simulink model "passband_filter_2023b"  (R2023b)
settings: Solver=VariableStepAuto  StartTime=0.0  StopTime=10.768  RelTol=1e-3
values from neighbouring files (symbols this model uses):
  den = den{1}    [Km_con_filtri.m]    (also in fft_signal_analysis.m)
  den2 = den2{1}    [Km_con_filtri.m]    (also in fft_signal_analysis.m)
  num = num{1}    [Km_con_filtri.m]    (also in fft_signal_analysis.m)
  num2 = num2{1}    [Km_con_filtri.m]    (also in fft_signal_analysis.m)
settings Model: Creator=riccardoorlandi  LastModifiedBy=lollo
settings RTWCC: GPUComputeCapability=5.0

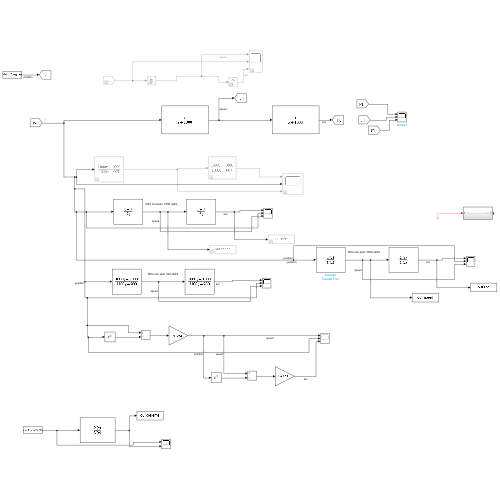
[thumbnail: Simulink's stored preview of the top-level diagram]
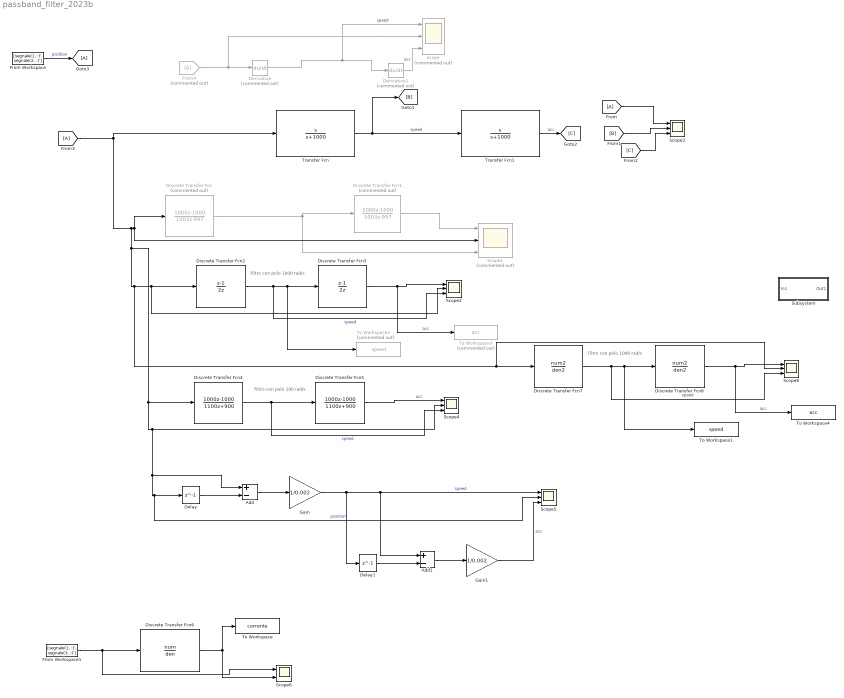
== system passband_filter_2023b ==
  note: filtro con polo 100 rad/s
  note: filtro con polo 1000 rad/s
  note: filtro con polo 1000 rad/s
  Add : Sum  Inputs=+-
  Add1 : Sum  Inputs=+-
  Delay : Delay  DelayLength=1
  Delay1 : Delay  DelayLength=1
  Derivative : Derivative  Commented=on
  Derivative1 : Derivative  Commented=on
  Discrete Transfer Fcn : DiscreteTransferFcn  Commented=on  Numerator=[1000 -1000]  Denominator=[1003 -997]
  Discrete Transfer Fcn1 : DiscreteTransferFcn  Commented=on  Numerator=[1000 -1000]  Denominator=[1003 -997]
  Discrete Transfer Fcn2 : DiscreteTransferFcn  Numerator=[1 -1]  Denominator=[2 0]
  Discrete Transfer Fcn3 : DiscreteTransferFcn  Numerator=[1 -1]  Denominator=[2 0]
  Discrete Transfer Fcn4 : DiscreteTransferFcn  Numerator=[1000 -1000]  Denominator=[1100 900]
  Discrete Transfer Fcn5 : DiscreteTransferFcn  Numerator=[1000 -1000]  Denominator=[1100 900]
  Discrete Transfer Fcn6 : DiscreteTransferFcn  Numerator=num  Denominator=den
  Discrete Transfer Fcn7 : DiscreteTransferFcn  Numerator=num2  Denominator=den2
  Discrete Transfer Fcn8 : DiscreteTransferFcn  Numerator=num2  Denominator=den2
  From : From
  From Workspace : FromWorkspace  VariableName=[segnale(1, :)', segnale(2, :)']  SampleTime=0.002
  From Workspace1 : FromWorkspace  VariableName=[segnale(1, :)', segnale(3, :)']  SampleTime=0.002
  From3 : From
  From4 : From  Commented=on
  Gain : Gain  Gain=1/0.002
  Gain1 : Gain  Gain=1/0.002
  Goto3 : Goto
  Scope : Scope  Commented=on  NumInputPorts=3
  Scope1 : Scope  Commented=on  NumInputPorts=3
  Scope{2..5,8} (5 alike) : Scope  NumInputPorts=3
  Scope6 : Scope  NumInputPorts=2
  Subsystem : Subsystem
  To Workspace : ToWorkspace  VariableName=corrente  SampleTime=-1
      settings: Save2DSignal=2-D array (concatenate along first dimension)
  To Workspace1 : ToWorkspace  VariableName=speed  SampleTime=-1
      settings: Save2DSignal=2-D array (concatenate along first dimension)
  To Workspace2 : ToWorkspace  Commented=on  VariableName=speed  SampleTime=-1
      settings: Save2DSignal=2-D array (concatenate along first dimension)
  To Workspace3 : ToWorkspace  Commented=on  VariableName=acc  SampleTime=-1
      settings: Save2DSignal=2-D array (concatenate along first dimension)
  To Workspace4 : ToWorkspace  VariableName=acc  SampleTime=-1
      settings: Save2DSignal=2-D array (concatenate along first dimension)
  Transfer Fcn : TransferFcn  Numerator=[1 0]  Denominator=[1 1000]
  Transfer Fcn1 : TransferFcn  Numerator=[1 0]  Denominator=[1 1000]
  wires:
  Transfer Fcn/1 -> [B], Transfer Fcn1/1  "speed"
  Transfer Fcn1/1 -> [C]  "acc"
  From/1 -> Scope3/1
  [B] -> Scope3/2
  [C] -> Scope3/3
  Derivative/1 -> Scope/1, Derivative1/1  "speed"
  Derivative1/1 -> Scope/3  "acc"
  Discrete Transfer Fcn/1 -> Scope1/3, Discrete Transfer Fcn1/1
  Discrete Transfer Fcn1/1 -> Scope1/1
  Discrete Transfer Fcn2/1 -> Scope2/3, To Workspace2/1, Discrete Transfer Fcn3/1  "speed"
  Discrete Transfer Fcn3/1 -> To Workspace3/1, Scope2/1  "acc"
  Discrete Transfer Fcn5/1 -> Scope4/1  "acc"
  Discrete Transfer Fcn4/1 -> Scope4/3, Discrete Transfer Fcn5/1  "speed"
  Delay/1 -> Add/2
  Add/1 -> Gain/1
  Delay1/1 -> Add1/2
  Add1/1 -> Gain1/1
  Gain/1 -> Delay1/1, Add1/1, Scope5/1  "speed"
  Gain1/1 -> Scope5/3  "acc"
  From Workspace1/1 -> Scope6/1, Discrete Transfer Fcn6/1
  Discrete Transfer Fcn6/1 -> To Workspace/1, Scope6/2
  From3/1 -> Add/1, Scope5/2, Delay/1, Scope4/2, Discrete Transfer Fcn4/1, Scope8/2, Discrete Transfer Fcn7/1, Scope2/2, Discrete Transfer Fcn2/1, Scope1/2, Discrete Transfer Fcn/1, Transfer Fcn/1  "position"
  Discrete Transfer Fcn7/1 -> Scope8/3, To Workspace1/1, Discrete Transfer Fcn8/1  "speed"
  Discrete Transfer Fcn8/1 -> To Workspace4/1, Scope8/1  "acc"
  From Workspace/1 -> Goto3/1  "position"
  From4/1 -> Scope/2, Derivative/1
  ? -> Subsystem/1(In1)

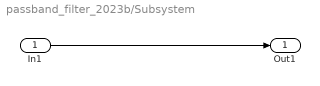
== system passband_filter_2023b/Subsystem ==
  In1 : Inport
  Out1 : Outport
  wires:
  In1/1 -> Out1/1
